simulink model "PROJET_PSC_MAX"  (R2019b)
settings: Solver=FixedStepAuto  StartTime=0.0  StopTime=10  RelTol=1e-3
values from neighbouring files (symbols this model uses):
  Nb_pilotes = Nb_pilotes+1    (= 26)    [script_result_test.m]
  Nb_porteuses_max = double(uint32(Temps_symbole*Bande_disponible))    [script_result_test.m]
  Nb_porteuses_utiles = double(uint32(Nb_porteuses_max - Nb_pilotes))    [script_result_test.m]
  Output_buffer = Taille_du_prefixe_cyclique+Puissance_de_2    [script_result_test.m]
  Puissance_de_2 = 2^la_puissance    (= 1)    [script_result_test.m]
  RCV_delay_ERC = Nb_porteuses_utiles*2    [script_result_test.m]
  Sample_Tps = Temps_symbole /(2*Nb_porteuses_utiles)    [script_result_test.m]
  Taille_du_prefixe_cyclique = ceil(Puissance_de_2/coef) + 10    [script_result_test.m]
undefined symbols (not defined in the file or in its folder): doppler
libraries: simulink x12, dspindex x8, commsink2 x6, dspxfrm3 x2, commdigbbndpm3 x2, commchan3 x2, commrandsrc3 x1
settings Model: SimulationMode=accelerator  Creator=adamb  LastModifiedBy=adamb

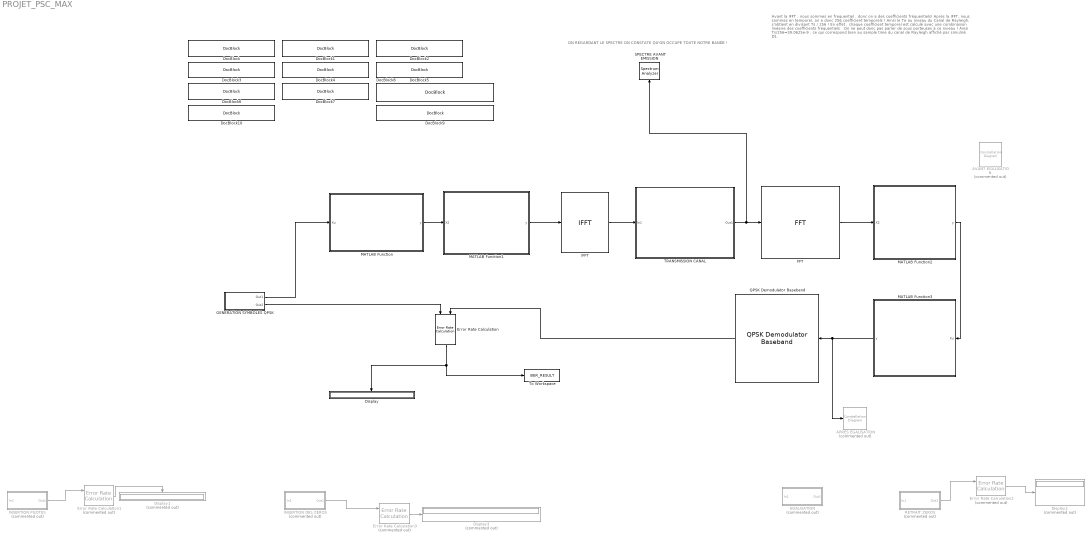
== system PROJET_PSC_MAX ==
  note: Avant la IFFT , nous sommes en frequentiel , donc on a des coefficients fréquentiels!
      | Après la IFFT, nous sommes en temporel, on a donc 256 coefficient temporels !
      | Ainsi le Te au niveau du Canal de Rayleigh, s'obtient en divisant Ts / 256 ! En effet , chaque coefficient temporel est calculé avec une combinaison linéaire des coefficients fréquentiels . On ne peut donc pas parler de sous porteuses à ce niveau !
      |
      | Ainsi Ts/256=39.0625e-9 , ce qui correspond bien au sample time du canal de Rayleigh affiché par simulink D1.
  note: ON REGARDANT LE SPECTRE ON CONSTATE QU'ON OCCUPE TOUTE NOTRE BANDE !
  APRES EGALISATION : ConstellationDiagram  Commented=on
  AVANT EGALISATION : ConstellationDiagram  Commented=on
  Display : Display
  Display1 : Display  Commented=on
  Display2 : Display  Commented=on
  Display3 : Display  Commented=on
  DocBlock{,1..10} (11 alike) : simulink/Model-Wide Utilities/DocBlock  DocumentType=Text  mask(DocBlock){}
      content=|
      | Type your documentation here
      DocBlock mask Display:
      | % This is a new mask on top of the base mask.
      | % Use "View base mask" link below to see the base mask.
      | 
      | Bande_disponible = evalin('base', 'Bande_disponible');
      | fprintf(['Bande_disponible = ',num2str(Bande_disponible*1e-6),' MHz']);
      DocBlock1 mask Display:
      | % This is a new mask on top of the base mask.
      | % Use "View base mask" link below to see the base mask.
      | 
      | Tau_max = evalin('base', 'Tau_max');
      | fprintf(['Tau_max = ',num2str(Tau_max/1e-9),' ns']);
      DocBlock10 mask Display:
      | % This is a new mask on top of the base mask.
      | % Use "View base mask" link below to see the base mask.
      | 
      | Nb_de_zeros = evalin('base', 'Nb_de_zeros');
      | fprintf(['Nb_de_zeros = ',num2str(Nb_de_zeros)]);
      DocBlock2 mask Display:
      | % This is a new mask on top of the base mask.
      | % Use "View base mask" link below to see the base mask.
      | 
      | Temps_symbole = evalin('base', 'Temps_symbole');
      | fprintf(['Temps_symbole = ',num2str(Temps_symbole),' s']);
      DocBlock3 mask Display:
      | % This is a new mask on top of the base mask.
      | % Use "View base mask" link below to see the base mask.
      | 
      | Nb_porteuses_max = evalin('base', 'Nb_porteuses_max');
      | fprintf(['Nb_porteuses_max = ',num2str(Nb_porteuses_max)]);
      DocBlock4 mask Display:
      | % This is a new mask on top of the base mask.
      | % Use "View base mask" link below to see the base mask.
      | 
      | Nb_pilotes = evalin('base', 'Nb_pilotes');
      | fprintf(['Nb_pilotes = ',num2str(Nb_pilotes)]);
      DocBlock5 mask Display:
      | % This is a new mask on top of the base mask.
      | % Use "View base mask" link below to see the base mask.
      | 
      | Nb_porteuses_utiles = evalin('base', 'Nb_porteuses_utiles');
      | fprintf(['Nb_porteuses_utiles = ',num2str(Nb_porteuses_utiles)]);
      DocBlock6 mask Display:
      | % This is a new mask on top of the base mask.
      | % Use "View base mask" link below to see the base mask.
      | 
      | Taille_du_prefixe_cyclique = evalin('base', 'Taille_du_prefixe_cyclique');
      | fprintf(['Taille_du_prefixe_cyclique = ',num2str(Taille_du_prefixe_cyclique)]);
      DocBlock7 mask Display:
      | % This is a new mask on top of the base mask.
      | % Use "View base mask" link below to see the base mask.
      | 
      | Temps_echantillonnage = evalin('base', 'Temps_echantillonnage');
      | fprintf(['Temps_echantillonnage = ',num2str(Temps_echantillonnage/1e-9),' ns']);
      DocBlock8 mask Display:
      | % This is a new mask on top of the base mask.
      | % Use "View base mask" link below to see the base mask.
      | 
      | Vecteur_delay = evalin('base', 'Vecteur_delay');
      | fprintf(['Vecteur_delay = ',num2str(Vecteur_delay/1e-9),' ns']);
      DocBlock9 mask Display:
      | % This is a new mask on top of the base mask.
      | % Use "View base mask" link below to see the base mask.
      | 
      | Vecteur_de_Gain = evalin('base', 'Vecteur_de_Gain');
      | fprintf(['Vecteur_de_Gain = ',num2str(Vecteur_de_Gain),' dB']);
  EGALISATION : Subsystem  Commented=on
  Error Rate Calculation : commsink2/Error Rate Calculation  N=RCV_delay_ERC  st_delay=0  cp_mode=Entire frame  subframe=[]  PMode=Port  WsName=ErrorVec  RsMode2=off  stop=off  numErr=100  maxBits=1e6
      settings: SourceProductName=Communications Toolbox
  Error Rate Calculation1 : commsink2/Error Rate Calculation  Commented=on  N=0  st_delay=0  cp_mode=Entire frame  subframe=[]  PMode=Port  WsName=ErrorVec  RsMode2=off  stop=off  numErr=100  maxBits=1e6
      settings: SourceProductName=Communications Toolbox
  Error Rate Calculation2 : commsink2/Error Rate Calculation  Commented=on  N=0  st_delay=0  cp_mode=Entire frame  subframe=[]  PMode=Port  WsName=ErrorVec  RsMode2=off  stop=off  numErr=100  maxBits=1e6
      settings: SourceProductName=Communications Toolbox
  Error Rate Calculation3 : commsink2/Error Rate Calculation  Commented=on  N=0  st_delay=0  cp_mode=Entire frame  subframe=[]  PMode=Port  WsName=ErrorVec  RsMode2=off  stop=off  numErr=100  maxBits=1e6
      settings: SourceProductName=Communications Toolbox
  FFT : dspxfrm3/FFT  FFTImplementation=Auto  CompMethod=Table lookup  TableOpt=NEW  TableOptActive=Speed  BitRevOrder=off  Normalize=off  InheritFFTLength=on  FFTLength=64  WrapInput=on  roundingMode=Floor  overflowMode=off  firstCoeffDataTypeStr=Inherit: Same word length as input  firstCoeffLastDataTypeStr=Inherit: Same word length as input  outputMin=[]  outputMax=[]
  GENERATION SYMBOLES QPSK : Subsystem
  IFFT : dspxfrm3/IFFT  FFTImplementation=Auto  CompMethod=Table lookup  TableOpt=NEW  TableOptActive=Speed  BitRevOrder=off  cs_in=off  Normalize=on  InheritFFTLength=on  FFTLength=64  WrapInput=on  mode=Complex  outSamplingMode=Sample based  roundingMode=Floor  overflowMode=off  firstCoeffDataTypeStr=Inherit: Same word length as input  firstCoeffLastDataTypeStr=Inherit: Same word length as input  outputMin=[]  outputMax=[]
      settings: SourceProductName=DSP System Toolbox
  "INSERTION DES ZEROS " : Subsystem  Commented=on
  INSERTION PILOTES : Subsystem  Commented=on
  MATLAB Function : MATLAB Function  TreatAsAtomicUnit=on
  MATLAB Function1 : MATLAB Function  TreatAsAtomicUnit=on
  MATLAB Function2 : MATLAB Function  TreatAsAtomicUnit=on
  MATLAB Function3 : MATLAB Function  TreatAsAtomicUnit=on
  QPSK Demodulator Baseband : commdigbbndpm3/QPSK Demodulator Baseband  OutType=Bit  DecType=Hard decision  VarSource=Dialog  Variance=1  Dec=Gray  Ph=pi/4  outDtype1=Inherit via internal rule  outDtype2=Inherit via internal rule  derotateFactorWordLen=16  derotateFactorDataTypeStr=Inherit: Same word length as input  derotateFactorLastDataTypeStr=Inherit: Same word length as input
      settings: SourceProductName=Communications Toolbox
  RETRAIT ZEROS : Subsystem  Commented=on
  SPECTRE AVANT EMISSION : SpectrumAnalyzer
  TRANSMISSION CANAL : Subsystem
  To Workspace : ToWorkspace  VariableName=BER_RESULT  SampleTime=-1
      settings: Save2DSignal=2-D array (concatenate along first dimension)
  wires:
  MATLAB Function3/1(y) -> APRES EGALISATION/1, QPSK Demodulator Baseband/1
  Error Rate Calculation/1 -> Display/1, To Workspace/1
  GENERATION SYMBOLES QPSK/2(Out2) -> Error Rate Calculation/1
  QPSK Demodulator Baseband/1 -> Error Rate Calculation/2
  GENERATION SYMBOLES QPSK/1(Out1) -> MATLAB Function/1(Xu)
  INSERTION PILOTES/1(Out1) -> Error Rate Calculation1/1
  MATLAB Function1/1(y) -> IFFT/1
  Error Rate Calculation1/1 -> Display1/1
  FFT/1 -> MATLAB Function2/1(X2)
  RETRAIT ZEROS/1(Out1) -> Error Rate Calculation2/1
  MATLAB Function2/1(y) -> MATLAB Function3/1(Xu)
  Error Rate Calculation2/1 -> Display2/1
  Error Rate Calculation3/1 -> Display3/1
  "INSERTION DES ZEROS "/1(Out1) -> Error Rate Calculation3/1
  MATLAB Function/1(y) -> MATLAB Function1/1(X2)
  IFFT/1 -> TRANSMISSION CANAL/1(In1)
  TRANSMISSION CANAL/1(Out1) -> SPECTRE AVANT EMISSION/1, FFT/1

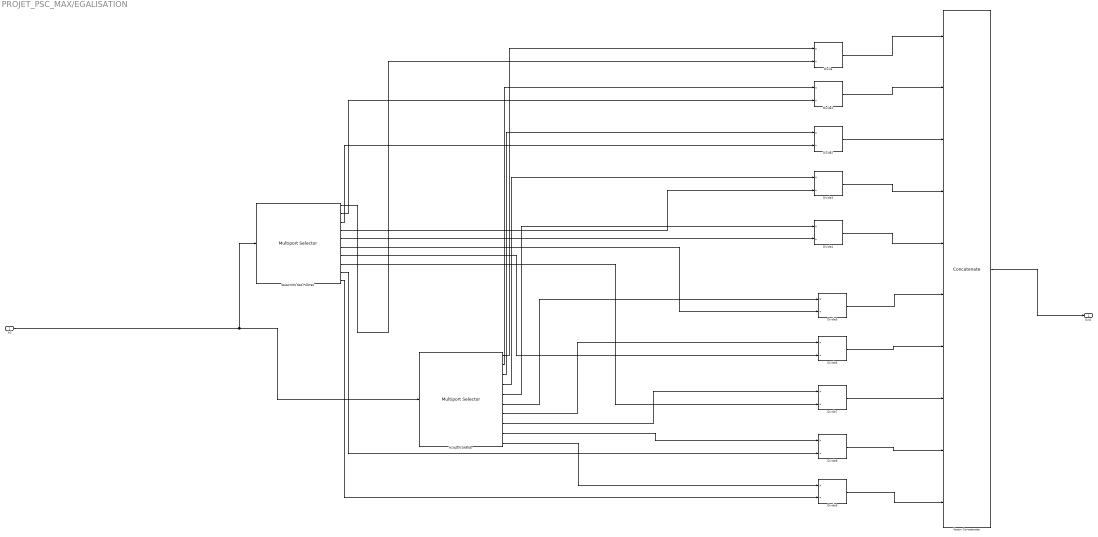
== system PROJET_PSC_MAX/EGALISATION ==
  In1 : Inport
  Divide{,1..9} (10 alike) : Product  Inputs=*/
  Multiport Selector : dspindex/Multiport Selector  rowsOrCols=Rows  idxCellArray={ [2:20], [22:40], [42:60], [62:80], [82:100], [102:120], [122:140], [142:160], [162:180], [182:200] }  idxErrMode=Clip Index
  "SELECTION DES PILOTES " : dspindex/Multiport Selector  rowsOrCols=Rows  idxCellArray={ [1],[21],[41],[61],[81],[101],[121],[141],[161],[181]}  idxErrMode=Clip Index
  Vector Concatenate : Concatenate  NumInputs=10
  Out1 : Outport
  wires:
  In1/1 -> Multiport Selector/1, "SELECTION DES PILOTES "/1
  "SELECTION DES PILOTES "/1 -> Divide/2
  Multiport Selector/10 -> Divide9/1
  Multiport Selector/9 -> Divide8/1
  Multiport Selector/8 -> Divide7/1
  Multiport Selector/7 -> Divide6/1
  Multiport Selector/6 -> Divide5/1
  Multiport Selector/5 -> Divide4/1
  Multiport Selector/4 -> Divide3/1
  Multiport Selector/3 -> Divide2/1
  Multiport Selector/2 -> Divide1/1
  Multiport Selector/1 -> Divide/1
  Divide/1 -> Vector Concatenate/1
  Divide1/1 -> Vector Concatenate/2
  Divide2/1 -> Vector Concatenate/3
  Divide3/1 -> Vector Concatenate/4
  Divide4/1 -> Vector Concatenate/5
  Divide5/1 -> Vector Concatenate/6
  Divide6/1 -> Vector Concatenate/7
  Divide7/1 -> Vector Concatenate/8
  Divide8/1 -> Vector Concatenate/9
  Divide9/1 -> Vector Concatenate/10
  Vector Concatenate/1 -> Out1/1
  "SELECTION DES PILOTES "/2 -> Divide1/2
  "SELECTION DES PILOTES "/3 -> Divide2/2
  "SELECTION DES PILOTES "/4 -> Divide3/2
  "SELECTION DES PILOTES "/5 -> Divide4/2
  "SELECTION DES PILOTES "/6 -> Divide5/2
  "SELECTION DES PILOTES "/7 -> Divide6/2
  "SELECTION DES PILOTES "/8 -> Divide7/2
  "SELECTION DES PILOTES "/9 -> Divide8/2
  "SELECTION DES PILOTES "/10 -> Divide9/2

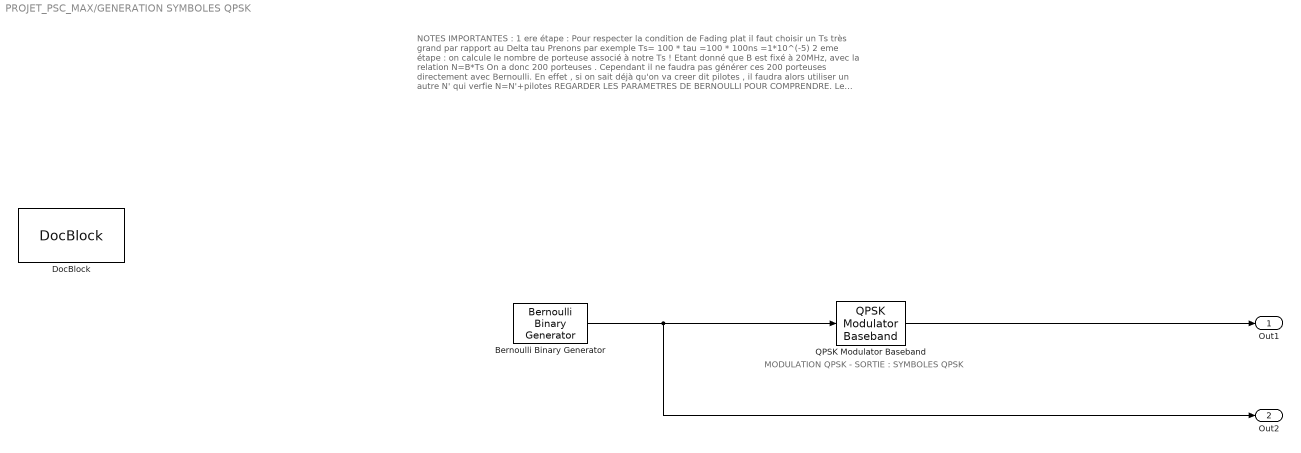
== system PROJET_PSC_MAX/GENERATION SYMBOLES QPSK ==
  note: MODULATION QPSK - SORTIE : SYMBOLES QPSK
  note: NOTES IMPORTANTES :
      |
      | 1 ere étape : Pour respecter la condition de Fading plat il faut choisir un Ts très grand par rapport au Delta tau
      |
      | Prenons par exemple Ts= 100 * tau =100 * 100ns =1*10^(-5)
      |
      | 2 eme étape : on calcule le nombre de porteuse associé à notre Ts !
      | Etant donné que B est fixé à 20MHz, avec la relation N=B*Ts
      | On a donc 200 porteuses .
      |
      | Cependant il ne faudra pas générer ces 200 porteuses directement avec Bernoulli. En effet , si on sait déjà qu'on va creer dit pilotes , il faudra alors utiliser un autre N' qui verfie N=N'+pilotes
      |
      | REGARDER LES PARAMETRES DE BERNOULLI POUR COMPRENDRE.
      |
      | Le sample time Tb s'obtient en calculant Ts/2N or comme on veut 10 pilotes qu'on va rajouter plus tard , il faut les retirer au debut du calcul sinon on agrandit notre bande .
  Bernoulli Binary Generator : commrandsrc3/Bernoulli Binary Generator  ProbabilityOfZero=0.5  SeedSource=Auto  Seed=0  SampleTime=Sample_Tps  SamplesPerFrame=Sample_rt  OutputDataType=double  SimulateUsing=Code generation
      settings: SourceProductName=Communications Toolbox
  DocBlock : simulink/Model-Wide Utilities/DocBlock  DocumentType=Text  mask(DocBlock){}
      content=|
      | Type your documentation here
      mask Display:
      | % This is a new mask on top of the base mask.
      | % Use "View base mask" link below to see the base mask.
      | 
      | coef = evalin('base', 'coef');
      | fprintf(['coef=',num2str(coef)]);
  QPSK Modulator Baseband : commdigbbndpm3/QPSK Modulator Baseband  InType=Bit  Enc=Gray  Ph=pi/4  outDtype=double  outWordLen=16  outUDDataType=sfix(16)  outFracLenMode=Best precision  outFracLen=15  outDataTypeStr=double  outLastDataTypeStr=double
      settings: SourceProductName=Communications Toolbox
  Out1 : Outport
  Out2 : Outport  Port=2
  wires:
  Bernoulli Binary Generator/1 -> Out2/1, QPSK Modulator Baseband/1
  QPSK Modulator Baseband/1 -> Out1/1

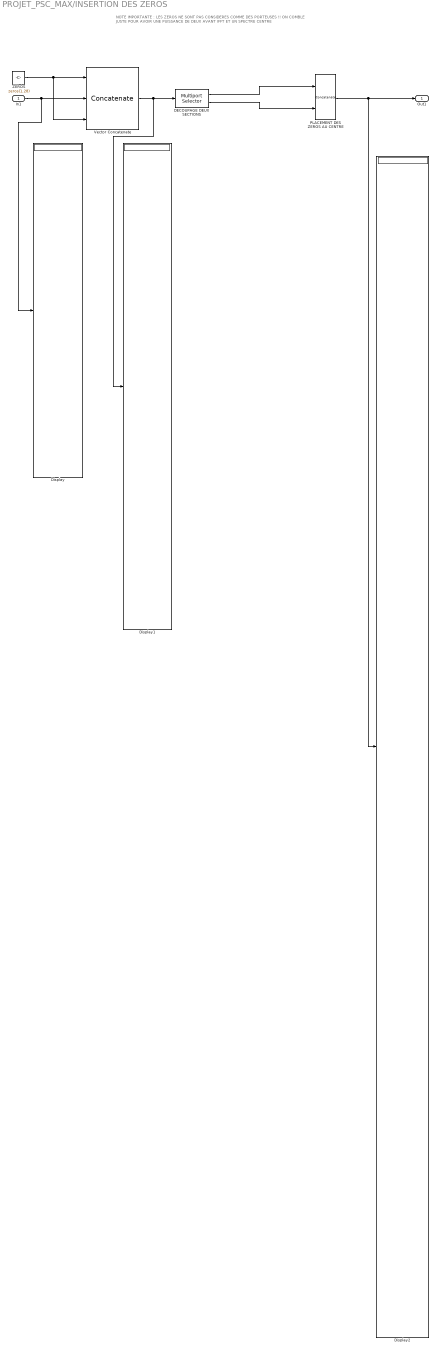
== system PROJET_PSC_MAX/INSERTION DES ZEROS  ==
  note: NOTE IMPORTANTE :
      |
      | LES ZEROS NE SONT PAS CONSIDERES COMME DES PORTEUSES !!
      | ON COMBLE JUSTE POUR AVOIR UNE PUISSANCE DE DEUX AVANT IFFT ET UN SPECTRE CENTRE
  In1 : Inport
  DECOUPAGE DEUX SECTIONS : dspindex/Multiport Selector  rowsOrCols=Rows  idxCellArray={ [129:256], [1:128]}  idxErrMode=Clip Index
  Display : Display
  Display1 : Display
  Display2 : Display
  PLACEMENT DES ZEROS AU CENTRE : Concatenate
  Vector Concatenate : Concatenate  NumInputs=3
  ZEROS : Constant  Value=zeros(1,28)
  Out1 : Outport
  wires:
  In1/1 -> Display/1, Vector Concatenate/2
  ZEROS/1 -> Vector Concatenate/3, Vector Concatenate/1
  Vector Concatenate/1 -> Display1/1, DECOUPAGE DEUX SECTIONS/1
  DECOUPAGE DEUX SECTIONS/1 -> PLACEMENT DES ZEROS AU CENTRE/1
  DECOUPAGE DEUX SECTIONS/2 -> PLACEMENT DES ZEROS AU CENTRE/2
  PLACEMENT DES ZEROS AU CENTRE/1 -> Display2/1, Out1/1

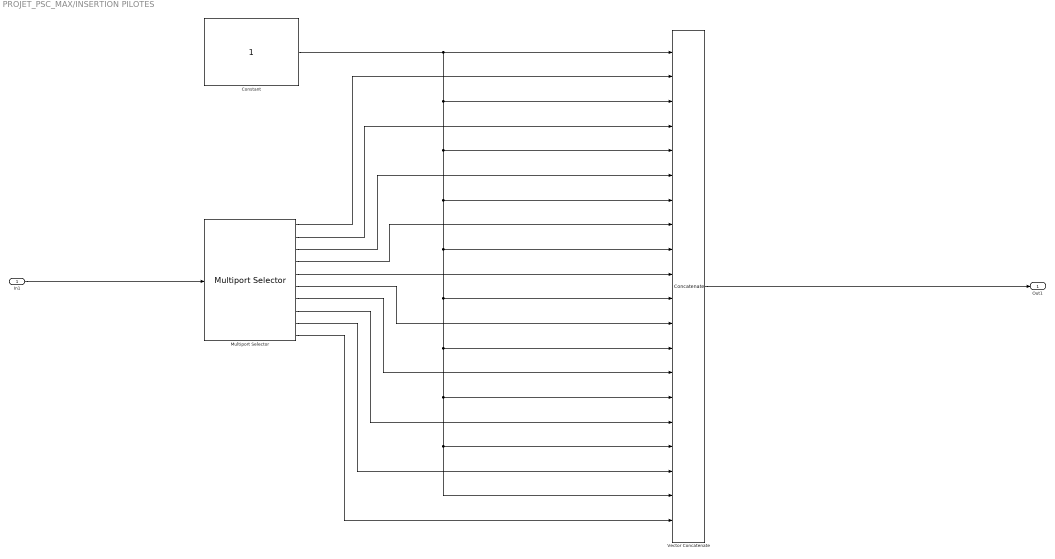
== system PROJET_PSC_MAX/INSERTION PILOTES ==
  In1 : Inport
  Constant : Constant
  Multiport Selector : dspindex/Multiport Selector  rowsOrCols=Rows  idxCellArray={ [1:19], [20:38], [39:57], [58:76], [77:95], [96:114], [115:133], [134:152], [153:171], [172:190] }  idxErrMode=Clip Index
  Vector Concatenate : Concatenate  NumInputs=20
  Out1 : Outport
  wires:
  In1/1 -> Multiport Selector/1
  Constant/1 -> Vector Concatenate/5, Vector Concatenate/7, Vector Concatenate/19, Vector Concatenate/17, Vector Concatenate/15, Vector Concatenate/13, Vector Concatenate/11, Vector Concatenate/9, Vector Concatenate/3, Vector Concatenate/1
  Multiport Selector/1 -> Vector Concatenate/2
  Multiport Selector/2 -> Vector Concatenate/4
  Multiport Selector/3 -> Vector Concatenate/6
  Multiport Selector/4 -> Vector Concatenate/8
  Multiport Selector/5 -> Vector Concatenate/10
  Multiport Selector/6 -> Vector Concatenate/12
  Multiport Selector/7 -> Vector Concatenate/14
  Multiport Selector/8 -> Vector Concatenate/16
  Multiport Selector/9 -> Vector Concatenate/18
  Multiport Selector/10 -> Vector Concatenate/20
  Vector Concatenate/1 -> Out1/1

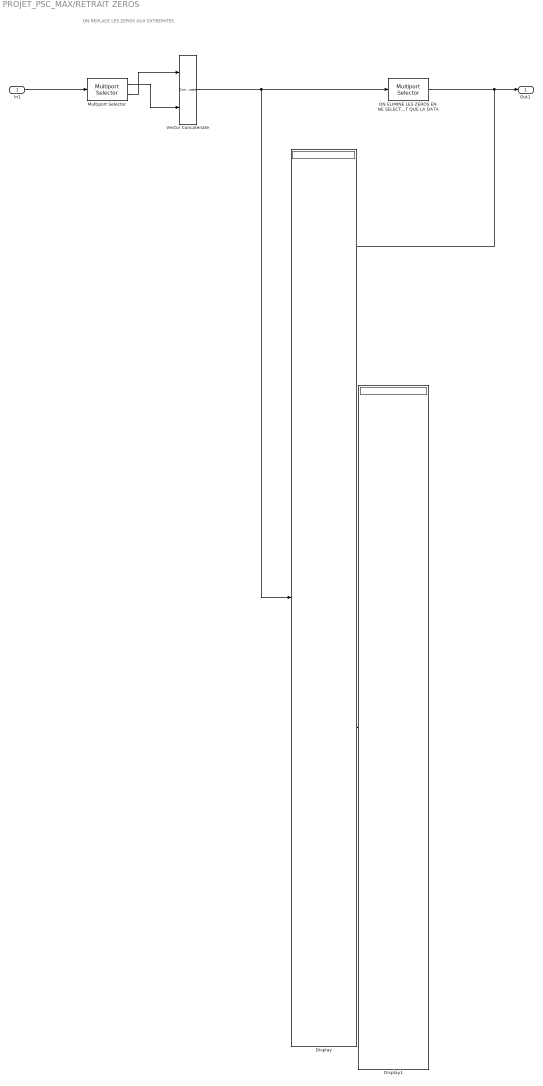
== system PROJET_PSC_MAX/RETRAIT ZEROS ==
  note: ON REPLACE LES ZEROS AUX EXTREMITES
  In1 : Inport
  Display : Display
  Display1 : Display
  Multiport Selector : dspindex/Multiport Selector  rowsOrCols=Rows  idxCellArray={ [1:128], [129:256],}  idxErrMode=Clip Index
  ON ELIMINE LES ZEROS EN NE SELECTIONNANT QUE LA DATA : dspindex/Multiport Selector  rowsOrCols=Rows  idxCellArray={ [29:228] }  idxErrMode=Clip Index
  Vector Concatenate : Concatenate
  Out1 : Outport
  wires:
  In1/1 -> Multiport Selector/1
  Vector Concatenate/1 -> Display/1, ON ELIMINE LES ZEROS EN NE SELECTIONNANT QUE LA DATA/1
  ON ELIMINE LES ZEROS EN NE SELECTIONNANT QUE LA DATA/1 -> Display1/1, Out1/1
  Multiport Selector/1 -> Vector Concatenate/2
  Multiport Selector/2 -> Vector Concatenate/1

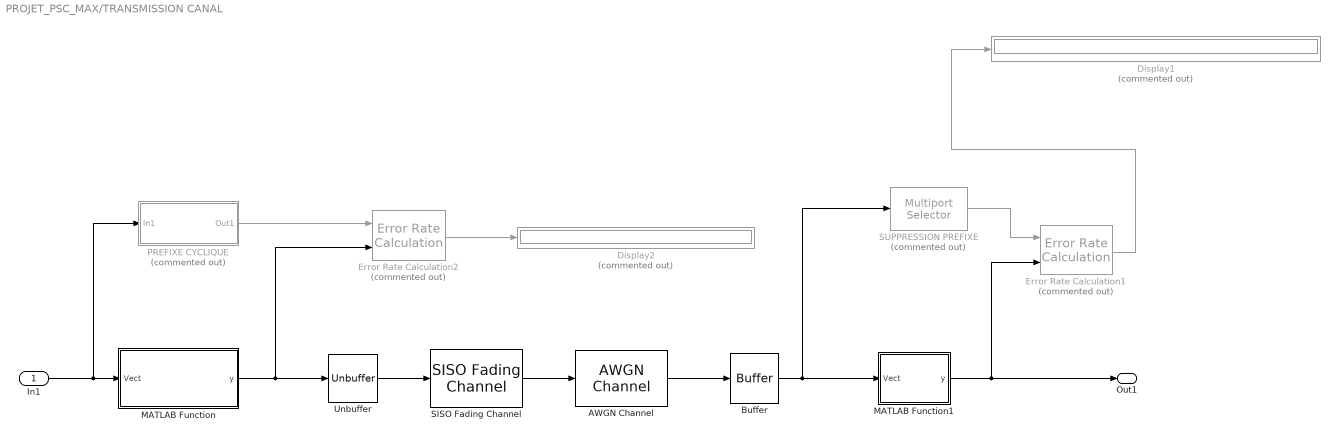
== system PROJET_PSC_MAX/TRANSMISSION CANAL ==
  In1 : Inport
  AWGN Channel : commchan3/AWGN Channel  InputProcessing=Columns as channels (frame based)  seed=67  noiseMode="Signal to noise ratio  (SNR)"  EbNodB=10  EsNodB=10  SNRdB=SNR_value  bitsPerSym=1  Ps=2e-3  Tsym=1  variance=1
      settings: SourceProductName=Communications Toolbox
  Buffer : Buffer  N=Output_buffer  OutputFrames=off
  Display1 : Display  Commented=on
  Display2 : Display  Commented=on
  Error Rate Calculation1 : commsink2/Error Rate Calculation  Commented=on  N=0  st_delay=0  cp_mode=Entire frame  subframe=[]  PMode=Port  WsName=ErrorVec  RsMode2=off  stop=off  numErr=100  maxBits=1e6
      settings: SourceProductName=Communications Toolbox
  Error Rate Calculation2 : commsink2/Error Rate Calculation  Commented=on  N=0  st_delay=0  cp_mode=Entire frame  subframe=[]  PMode=Port  WsName=ErrorVec  RsMode2=off  stop=off  numErr=100  maxBits=1e6
      settings: SourceProductName=Communications Toolbox
  MATLAB Function : MATLAB Function  TreatAsAtomicUnit=on
  MATLAB Function1 : MATLAB Function  TreatAsAtomicUnit=on
  PREFIXE CYCLIQUE : Subsystem  Commented=on
  SISO Fading Channel : commchan3/SISO Fading Channel  InheritSampleRate=on  SampleRate=1  PathDelays=Vecteur_delay  AveragePathGains=Vecteur_de_Gain  NormalizePathGains=on  FadingDistribution=Rayleigh  KFactor=3  DirectPathDopplerShift=0  DirectPathInitialPhase=0  MaximumDopplerShift=100  DopplerSpectrum=doppler('Jakes')  RandomStream=mt19937ar with seed  Seed=50  PathGainsOutputPort=off  ChannelFilterDelayOutputPort=off  SimulateUsing=Code generation  Visualization=Off  PathsForDopplerDisplay=1  SamplesToDisplay=25%
      settings: SourceProductName=Communications Toolbox
  SUPPRESSION PREFIXE : dspindex/Multiport Selector  Commented=on  rowsOrCols=Rows  idxCellArray={ [11:266] }  idxErrMode=Clip Index
  Unbuffer : Unbuffer
  Out1 : Outport
  wires:
  In1/1 -> PREFIXE CYCLIQUE/1(In1), MATLAB Function/1(Vect)
  Buffer/1 -> MATLAB Function1/1(Vect), SUPPRESSION PREFIXE/1
  Unbuffer/1 -> SISO Fading Channel/1
  SISO Fading Channel/1 -> AWGN Channel/1
  MATLAB Function/1(y) -> Error Rate Calculation2/2, Unbuffer/1
  Error Rate Calculation2/1 -> Display2/1
  PREFIXE CYCLIQUE/1(Out1) -> Error Rate Calculation2/1
  MATLAB Function1/1(y) -> Error Rate Calculation1/2, Out1/1
  Error Rate Calculation1/1 -> Display1/1
  SUPPRESSION PREFIXE/1 -> Error Rate Calculation1/1
  AWGN Channel/1 -> Buffer/1

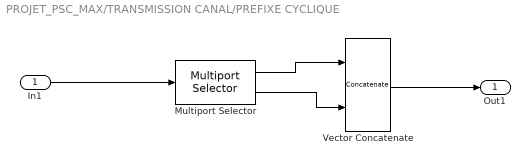
== system PROJET_PSC_MAX/TRANSMISSION CANAL/PREFIXE CYCLIQUE ==
  In1 : Inport
  Multiport Selector : dspindex/Multiport Selector  rowsOrCols=Rows  idxCellArray={[247:256],[1:256] }  idxErrMode=Clip Index
  Vector Concatenate : Concatenate
  Out1 : Outport
  wires:
  Multiport Selector/1 -> Vector Concatenate/1
  Multiport Selector/2 -> Vector Concatenate/2
  Vector Concatenate/1 -> Out1/1
  In1/1 -> Multiport Selector/1

== matlab function PROJET_PSC_MAX/MATLAB Function1 ==
  data: X2 input; y output; Nb_de_zeros parameter
function y = ADDING_ZEROS(X2, Nb_de_zeros)


%cela suppose que la longueur de X2 est paire !!!
if(Nb_de_zeros==0)
    RES=X2;
else
    if( mod(Nb_de_zeros,2)==0)
        B_1=zeros(1,Nb_de_zeros/2);

        X_2_1=X2(1:(length(X2)/2));
        X_2_2=X2((length(X2)/2)+1:length(X2));

        P_1=[X_2_2.' B_1];
        P_2=[B_1 X_2_1.'];
    end

    RES=[P_1 P_2].';
    
end
    
 
    
    
y = RES;

== matlab function PROJET_PSC_MAX/MATLAB Function ==
  data: Xu input; y output; Nb_pilotes parameter; Nb_porteuses_utiles parameter; Nb_porteuses_max parameter
function y = INSERTION_PILOTES(Xu, Nb_pilotes, Nb_porteuses_utiles, Nb_porteuses_max)



if(Nb_pilotes == 0)
    RES2=Xu;
    
else
    
    M=complex(zeros(Nb_pilotes,(Nb_porteuses_max/Nb_pilotes)));
    step=Nb_porteuses_utiles/Nb_pilotes;
    start=1;
    stop=step;
    for i=1:Nb_pilotes    
        M(i,1)=complex(1);
    end

    for k=1:Nb_pilotes
        C=2;
        for l=start:stop        
            M(k,C)=Xu(l);
            C=C+1;
        end
        start=start+step;
        stop=stop+step;
    end

    RES=M';
    RES2=conj(RES(:));
end




y = RES2;

== matlab function PROJET_PSC_MAX/MATLAB Function2 ==
  data: X2 input; y output; Nb_de_zeros parameter
function y = REMOVING_ZEROS(X2, Nb_de_zeros)


%cela suppose que la longueur de X2 est paire !!!

if(Nb_de_zeros==0)
    RES=X2;
else

    if( mod(Nb_de_zeros,2)==0)
        P_1=X2(1:(length(X2)/2));
        P_2=flip(X2((length(X2)/2)+1:length(X2)));

        V_1=P_1(1:(length(P_1)-(Nb_de_zeros/2)));
        V_2=flip(P_2(1:(length(P_2)-(Nb_de_zeros/2))));



    end

        RES=[V_2.' V_1.'].';
        
end
    
 
    
    
y = RES;

== matlab function PROJET_PSC_MAX/MATLAB Function3 ==
  data: Xu input; y output; Nb_pilotes parameter; Nb_porteuses_utiles parameter
function y = EGALISATION(Xu, Nb_pilotes, Nb_porteuses_utiles)

if(Nb_pilotes == 0)
    RES2=Xu;
    
else
  
    M=reshape(Xu,[],Nb_pilotes).';
    step=Nb_porteuses_utiles/Nb_pilotes;

    for k=1:Nb_pilotes-1
        poids_1=step-1;
        poids_2=1;
        for n=2:step+1        
            M(k,n)=M(k,n)/((poids_1/step)*M(k,1)+(poids_2/step)*M(k+1,1));
            poids_1=poids_1-1;
            poids_2=poids_2+1;
        end    
    end

    for n=2:step+1
        M(Nb_pilotes,n)=M(Nb_pilotes,n)/M(Nb_pilotes,1);
    end

    RES=M(:,2:step+1).'; %pour retire la première colonne qui contient tous les pilotes 

    RES2=RES(:);
    
    
end




y = RES2;

== matlab function PROJET_PSC_MAX/TRANSMISSION CANAL/MATLAB Function ==
  data: Vect input; y output; Taille_du_prefixe_cyclique parameter; Puissance_de_2 parameter
function y = INSERTION_PC(Vect, Taille_du_prefixe_cyclique, Puissance_de_2)

Start=Puissance_de_2+1-Taille_du_prefixe_cyclique;
P_C=Vect(Start:Puissance_de_2);
RES=[P_C.' Vect.'];

y = RES.';

== matlab function PROJET_PSC_MAX/TRANSMISSION CANAL/MATLAB Function1 ==
  data: Vect input; y output; Taille_du_prefixe_cyclique parameter; Puissance_de_2 parameter
function y = REMOVE_PC(Vect, Taille_du_prefixe_cyclique, Puissance_de_2)

RES=Vect(Taille_du_prefixe_cyclique+1:(Puissance_de_2+Taille_du_prefixe_cyclique));

y = RES;
